simulink model "DrivetrainTemplate_r2019b"  (R2021b)
settings: Solver=ode4  StartTime=0.0  StopTime=116  FixedStep=0.001  MaxStep=0.1  RelTol=1e-8  AbsTol=1e-7  EnableMultiTasking=on
InitFcn:
  | DrivetrainParameters;
values from neighbouring files (symbols this model uses):
  Ad = 0.019    [DrivetrainParameters.m]
  b_clu = 0.01    [DrivetrainParameters.m]
  Bd = 0.00004    (= 4e-05)    [DrivetrainParameters.m]
  clu_Fmax = 1825    [DrivetrainParameters.m]
  clu_Fn = [0 0 0 54 213 502 958 1232 1701 1850 1853]    [DrivetrainParameters.m]
  clu_pos = [0 23 45 65 87 109 125 143 168 182 201]    [DrivetrainParameters.m]
  clu_W0 = eng_W0    (= 5000)    [DrivetrainParameters.m]
  Fc = 1    [DrivetrainParameters.m]
  Fs = 1.5    [DrivetrainParameters.m]
  g = 9.81    [DrivetrainParameters.m]
  Je = 0.14+0.0295    (= 0.1695)    [DrivetrainParameters.m]
  Jw = 0.08474    [DrivetrainParameters.m]
  m_veh = 1428    [DrivetrainParameters.m]
  mu_k = 0.62    [DrivetrainParameters.m]
  n_max = 6900    [DrivetrainParameters.m]
  r_clu = 0.1035    [DrivetrainParameters.m]
  r_tyr = 0.3072    [DrivetrainParameters.m]
  sigma_0 = 10000    [DrivetrainParameters.m]
  sigma_1 = sqrt(10^5)    [DrivetrainParameters.m]
  T = [ ... (first row only)    [DrivetrainParameters.m]
  vs = 0.001    [DrivetrainParameters.m]
  whl_W0 = veh_V0/r_tyr    (= 102.177372685)    [DrivetrainParameters.m]
libraries: simulink x3
settings Model: Creator=bamason2  LastModifiedBy=byronmason
settings SolverCC: AutoScaleAbsTol=off  AlgebraicLoopSolver=TrustRegion
settings DataIOCC: SaveFormat=Array  SaveOutput=off  SaveTime=off  ReturnWorkspaceOutputs=off  SignalLoggingName=sigsOut
settings OptimizationCC: BooleanDataType=off  InitFltsAndDblsToZero=on  LifeSpan=inf
settings DebuggingCC: SaveWithParameterizedLinksMsg=none  UnderspecifiedInitializationDetection=Classic  MergeDetectMultiDrivingBlocksExec=none  SignalResolutionControl=TryResolveAllWithWarning  MultiTaskDSMMsg=warning  MultiTaskCondExecSysMsg=none  SFUnexpectedBacktrackingDiag=warning  SFNoUnconditionalDefaultTransitionDiag=warning  SFExecutionAtInitializationDiag=none  SFMachineParentedDataDiag=warning  ArithmeticOperatorsInVariantConditions=warning
settings HardwareCC: ProdBitPerPointer=32  ProdBitPerSizeT=32  ProdBitPerPtrDiffT=32  ProdLargestAtomicFloat=None  ProdIntDivRoundTo=Undefined  ProdEndianess=Unspecified  ProdWordSize=32  ProdHWDeviceType=32-bit Generic  TargetUnknown=on
settings ModelReferenceCC: PropagateSignalLabelsOutOfModel=off
settings SFSimCC: SimUseLocalCustomCode=off  CustomCodeUndefinedFunction=UseInterfaceOnly
settings RTWCC: RTWUseLocalCustomCode=off
settings CodeAppCC: StateflowObjectComments=on
settings GRTTargetCC: TargetFcnLib=ansi_tfl_tmw.mat  TargetLangStandard=C89/C90 (ANSI)  CombineOutputUpdateFcns=off  GRTInterface=on
settings ConfigComp: CovMetricSettings=dw  CovSaveCumulativeToWorkspaceVar=on  CovSaveSingleToWorkspaceVar=on  CovExternalEMLEnable=off

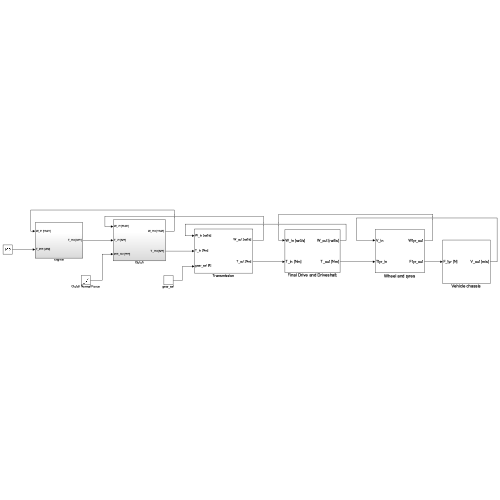
[thumbnail: Simulink's stored preview of the top-level diagram]
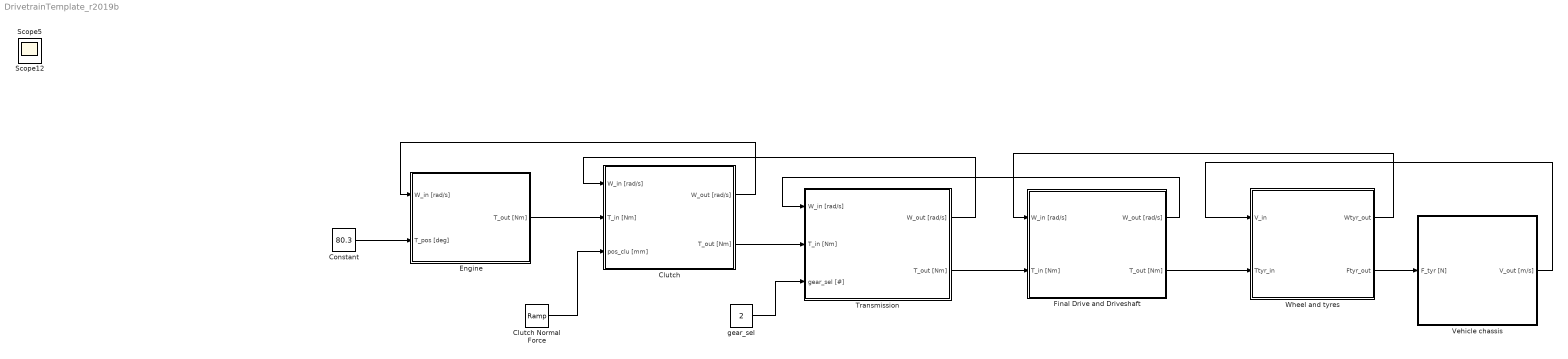
== system DrivetrainTemplate_r2019b ==
  Clutch : Subsystem
  Clutch Normal Force : simulink/Sources/Ramp  slope=clu_Fmax  start=clu_engage  InitialOutput=0
  Constant : Constant  Value=80.3
  Engine : Subsystem
  Final Drive and Driveshaft : Subsystem
  Transmission : Subsystem
  Vehicle chassis : Subsystem
  Wheel and tyres : Subsystem
  gear_sel : Constant  Value=2
  Scope12 : Scope
  Scope5 : Scope
  wires:
  Vehicle chassis/1(V_out [m/s]) -> Wheel and tyres/1(V_in)
  Transmission/2(T_out [Nm]) -> Final Drive and Driveshaft/2(T_in [Nm])
  gear_sel/1 -> Transmission/3(gear_sel [#])
  Final Drive and Driveshaft/1(W_out [rad/s]) -> Transmission/1(W_in [rad/s])
  Final Drive and Driveshaft/2(T_out [Nm]) -> Wheel and tyres/2(Ttyr_in)
  Clutch/2(T_out [Nm]) -> Transmission/2(T_in [Nm])
  Transmission/1(W_out [rad/s]) -> Clutch/1(W_in [rad/s])
  Clutch/1(W_out [rad/s]) -> Engine/1(W_in [rad/s])
  Constant/1 -> Engine/2(T_pos [deg])
  Engine/1(T_out [Nm]) -> Clutch/2(T_in [Nm])
  Wheel and tyres/1(Wtyr_out) -> Final Drive and Driveshaft/1(W_in [rad/s])
  Wheel and tyres/2(Ftyr_out) -> Vehicle chassis/1(F_tyr [N])
  Clutch Normal Force/1 -> Clutch/3(pos_clu [mm])

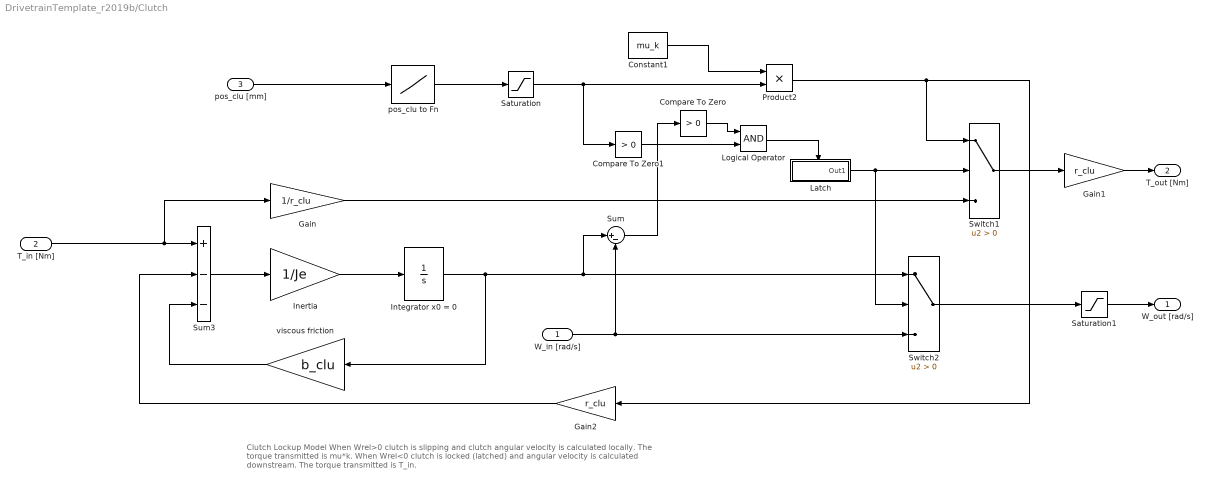
== system DrivetrainTemplate_r2019b/Clutch ==
  note: Clutch Lockup Model
      | When Wrel>0 clutch is slipping and clutch angular velocity is calculated locally. The torque transmitted
      | is mu*k.
      |
      | When Wrel<0 clutch is locked (latched) and angular velocity is calculated downstream. The torque transmitted
      | is T_in.
  W_in [rad/s] : Inport
  T_in [Nm] : Inport  Port=2
  pos_clu [mm] : Inport  Port=3
  Compare To Zero : simulink/Logic and Bit Operations/Compare To Zero  relop=>  OutDataTypeStr=boolean
  Compare To Zero1 : simulink/Logic and Bit Operations/Compare To Zero  relop=>  OutDataTypeStr=boolean
  Constant1 : Constant  Value=mu_k
  Gain : Gain  Gain=1/r_clu
  Gain1 : Gain  Gain=r_clu
  Gain2 : Gain  Gain=r_clu
  Inertia : Gain  Gain=1/Je  SaturateOnIntegerOverflow=on  OutDataTypeStr=Inherit: Same as input  ParamDataTypeStr=Inherit: Same as input
  Integrator x0 = 0 : Integrator  InitialCondition=clu_W0
  Latch : Subsystem  TreatAsAtomicUnit=on
  Logical Operator : Logic  AllPortsSameDT=off  OutDataTypeStr=boolean
  Product2 : Product
  Saturation : Saturate  UpperLimit=clu_Fmax  LowerLimit=0
  Saturation1 : Saturate  UpperLimit=6900/60*2*pi  LowerLimit=-inf
  Sum : Sum  Inputs=|+-
  Sum3 : Sum  Inputs=+--  InputSameDT=on  SaturateOnIntegerOverflow=on  OutDataTypeStr=Inherit: Same as first input
  Switch1 : Switch  Criteria=u2 > Threshold  SaturateOnIntegerOverflow=on  InputSameDT=on
  Switch2 : Switch  Criteria=u2 > Threshold  SaturateOnIntegerOverflow=on  InputSameDT=on
  pos_clu to Fn : Lookup_n-D  NumberOfTableDimensions=1  BreakpointsForDimension1=clu_pos  Table=clu_Fn  InternalRulePriority=Speed  RndMeth=Simplest  InputSameDT=on
  viscous friction : Gain  Gain=b_clu  SaturateOnIntegerOverflow=on  OutDataTypeStr=Inherit: Same as input  ParamDataTypeStr=Inherit: Same as input
  W_out [rad/s] : Outport
  T_out [Nm] : Outport  Port=2
  wires:
  Sum3/1 -> Inertia/1
  Gain1/1 -> T_out [Nm]/1
  Inertia/1 -> Integrator x0 = 0/1
  T_in [Nm]/1 -> Gain/1, Sum3/1
  Gain/1 -> Switch1/3
  Constant1/1 -> Product2/1
  Saturation/1 -> Product2/2, Compare To Zero1/1
  viscous friction/1 -> Sum3/3
  W_in [rad/s]/1 -> Switch2/3, Sum/2
  Integrator x0 = 0/1 -> Switch2/1, Sum/1, viscous friction/1
  Gain2/1 -> Sum3/2
  Product2/1 -> Gain2/1, Switch1/1
  Switch1/1 -> Gain1/1
  Switch2/1 -> Saturation1/1
  Latch/1(Out1) -> Switch1/2, Switch2/2
  Saturation1/1 -> W_out [rad/s]/1
  Compare To Zero/1 -> Logical Operator/1
  Logical Operator/1 -> Latch/Trigger
  Sum/1 -> Compare To Zero/1
  Compare To Zero1/1 -> Logical Operator/2
  pos_clu to Fn/1 -> Saturation/1
  pos_clu [mm]/1 -> pos_clu to Fn/1

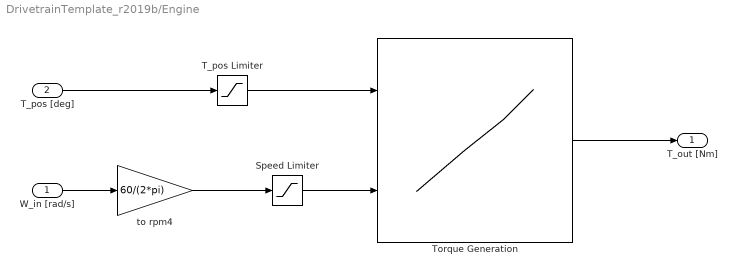
== system DrivetrainTemplate_r2019b/Engine ==
  W_in [rad/s] : Inport
  T_pos [deg] : Inport  Port=2
  Speed Limiter : Saturate  UpperLimit=n_max  LowerLimit=500
  T_pos Limiter : Saturate  UpperLimit=80.3  LowerLimit=0
  Torque Generation : Lookup2D  DialogController=Simulink.DDGSource  RowIndex=P  ColumnIndex=N  Table=T
  to rpm4 : Gain  Gain=60/(2*pi)  SaturateOnIntegerOverflow=on  OutDataTypeStr=Inherit: Same as input  ParamDataTypeStr=Inherit: Same as input
  T_out [Nm] : Outport
  wires:
  T_pos [deg]/1 -> T_pos Limiter/1
  W_in [rad/s]/1 -> to rpm4/1
  Torque Generation/1 -> T_out [Nm]/1
  to rpm4/1 -> Speed Limiter/1
  Speed Limiter/1 -> Torque Generation/2
  T_pos Limiter/1 -> Torque Generation/1

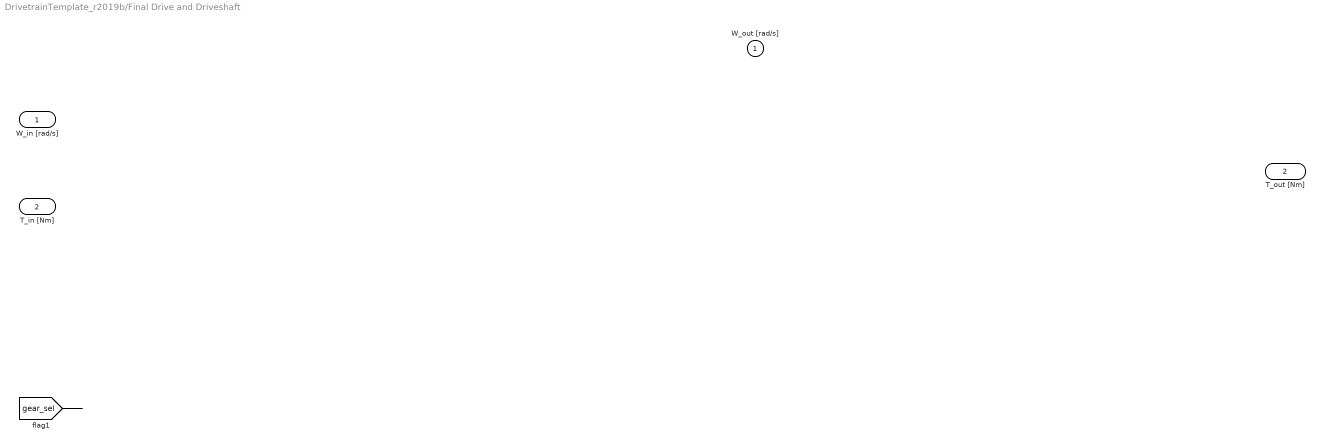
== system DrivetrainTemplate_r2019b/Final Drive and Driveshaft ==
  W_in [rad/s] : Inport
  T_in [Nm] : Inport  Port=2
  W_out [rad/s] : Outport
  T_out [Nm] : Outport  Port=2
  wires:
  [gear_sel] -> ?

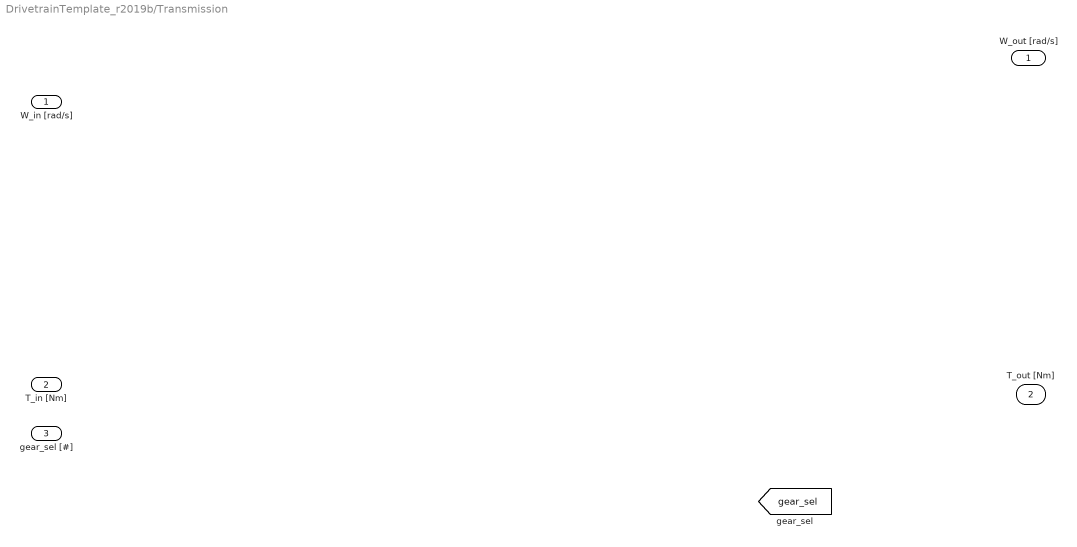
== system DrivetrainTemplate_r2019b/Transmission ==
  W_in [rad/s] : Inport
  T_in [Nm] : Inport  Port=2
  gear_sel [#] : Inport  Port=3
  W_out [rad/s] : Outport
  T_out [Nm] : Outport  Port=2
  tag scope: gear_sel=global

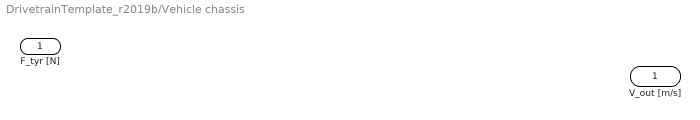
== system DrivetrainTemplate_r2019b/Vehicle chassis ==
  F_tyr [N] : Inport
  V_out [m/s] : Outport

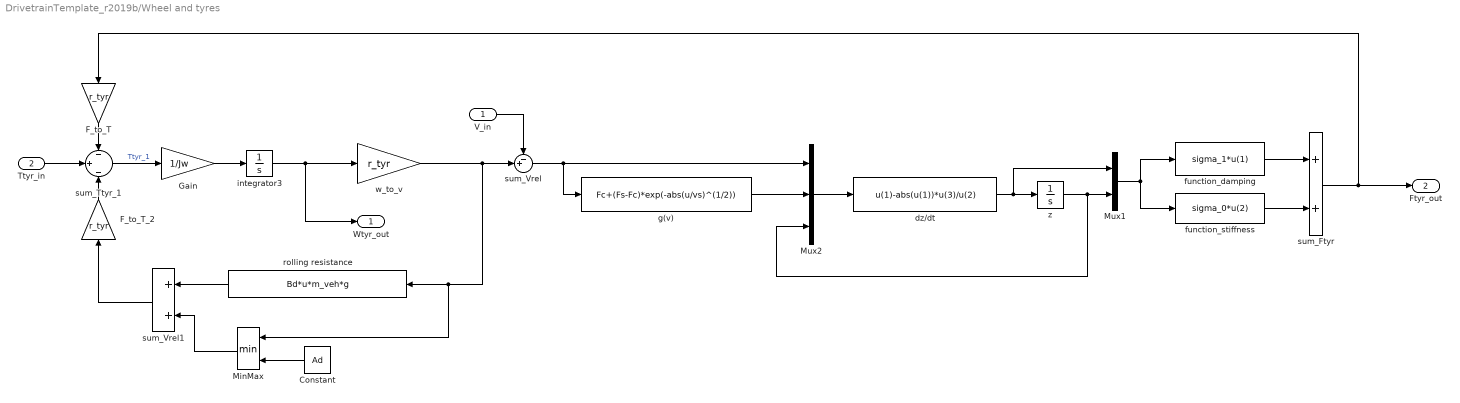
== system DrivetrainTemplate_r2019b/Wheel and tyres ==
  V_in : Inport
  Ttyr_in : Inport  Port=2
  Constant : Constant  Value=Ad
  F_to_T : Gain  Gain=r_tyr
  F_to_T_2 : Gain  Gain=r_tyr
  Gain : Gain  Gain=1/Jw
  MinMax : MinMax  Inputs=2
  Mux1 : Mux  Inputs=2
  Mux2 : Mux  Inputs=3
  dz/dt : Fcn  Expr=u(1)-abs(u(1))*u(3)/u(2)
  function_damping : Fcn  Expr=sigma_1*u(1)
  function_stiffness : Fcn  Expr=sigma_0*u(2)
  g(v) : Fcn  Expr=Fc+(Fs-Fc)*exp(-abs(u/vs)^(1/2))
  integrator3 : Integrator  InitialCondition=whl_W0
  rolling resistance : Fcn  Expr=Bd*u*m_veh*g
  sum_Ftyr : Sum
  sum_Ttyr_1 : Sum  Inputs=-|+|-
  sum_Vrel : Sum  Inputs=-+|  InputSameDT=on  SaturateOnIntegerOverflow=on  OutDataTypeStr=Inherit: Same as first input
  sum_Vrel1 : Sum  InputSameDT=on  SaturateOnIntegerOverflow=on  OutDataTypeStr=Inherit: Same as first input
  w_to_v : Gain  Gain=r_tyr
  z : Integrator  UpperSaturationLimit=1  LowerSaturationLimit=0
  Wtyr_out : Outport
  Ftyr_out : Outport  Port=2
  wires:
  w_to_v/1 -> sum_Vrel/2, MinMax/1, rolling resistance/1
  sum_Ttyr_1/1 -> Gain/1  "Ttyr_1"
  Gain/1 -> integrator3/1
  V_in/1 -> sum_Vrel/1
  Ttyr_in/1 -> sum_Ttyr_1/2
  Mux1/1 -> function_stiffness/1, function_damping/1
  rolling resistance/1 -> sum_Vrel1/1
  dz/dt/1 -> Mux1/1, z/1
  Mux2/1 -> dz/dt/1
  z/1 -> Mux2/3, Mux1/2
  g(v)/1 -> Mux2/2
  F_to_T/1 -> sum_Ttyr_1/1
  integrator3/1 -> Wtyr_out/1, w_to_v/1
  function_damping/1 -> sum_Ftyr/1
  function_stiffness/1 -> sum_Ftyr/2
  sum_Ftyr/1 -> F_to_T/1, Ftyr_out/1
  sum_Vrel/1 -> Mux2/1, g(v)/1
  F_to_T_2/1 -> sum_Ttyr_1/3
  MinMax/1 -> sum_Vrel1/2
  sum_Vrel1/1 -> F_to_T_2/1
  Constant/1 -> MinMax/2

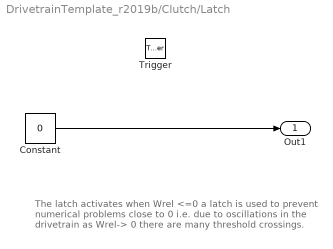
== system DrivetrainTemplate_r2019b/Clutch/Latch ==
  note: The latch activates when Wrel <=0 a latch is used to prevent
      | numerical problems close to 0 i.e. due to oscillations in the
      | drivetrain as Wrel-> 0  there are many threshold crossings.
  Trigger : TriggerPort  TriggerType=falling  VariantControl=(inherit)
  Constant : Constant  Value=0
  Out1 : Outport  InitialOutput=[1]
  wires:
  Constant/1 -> Out1/1
